simulink model "Impedance_with_fuzzy (1)"  (R2017b)
settings: Solver=ode45  StartTime=0.0  StopTime=20  RelTol=1e-3
libraries: cstblocks x1, fuzblock x1, simulink x1, commsrccod2 x1
settings Model: Creator=sansh  LastModifiedBy=pdesai24
settings CodeAppCC: StateflowObjectComments=on

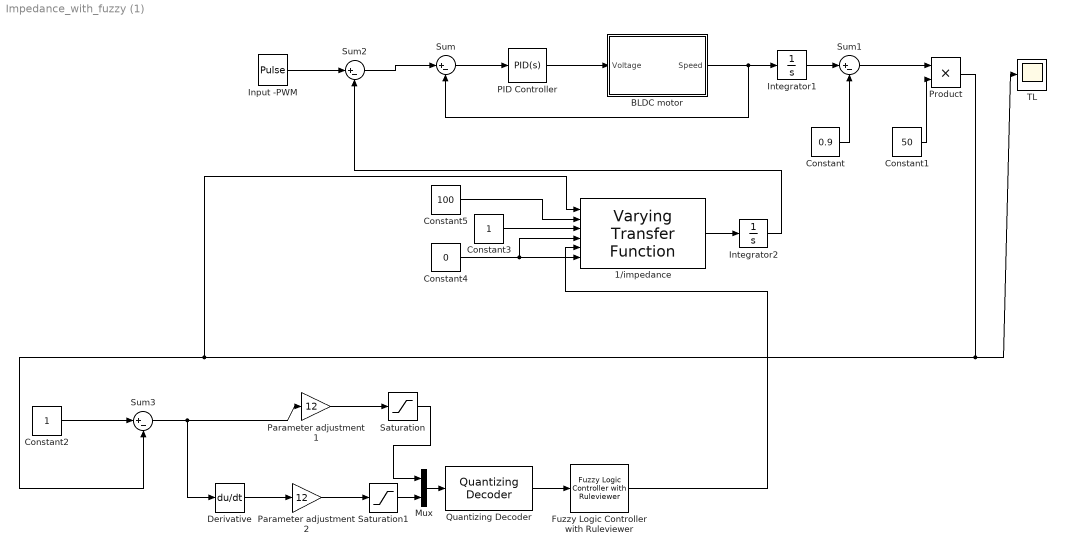
== system Impedance_with_fuzzy (1) ==
  1/impedance : cstblocks/Linear Parameter Varying/Varying Transfer Function  N=2
      settings: SourceProductName=Control System Toolbox
  BLDC motor : Subsystem
  Constant : Constant  Value=0.9
  Constant1 : Constant  Value=50
  Constant2 : Constant
  Constant3 : Constant
  Constant4 : Constant  Value=0
  Constant5 : Constant  Value=100
  Derivative : Derivative
  Fuzzy Logic Controller with Ruleviewer : fuzblock/Fuzzy Logic  Controller  with Ruleviewer  fismatrix=fuzzycntrl  Ts=2
  Input -PWM : DiscretePulseGenerator  PulseType=Time based  Amplitude=22  Period=10  PulseWidth=5  VectorParams1D=off
  Integrator1 : Integrator
  Integrator2 : Integrator
  Mux : Mux  Inputs=2
  PID Controller : simulink/Continuous/PID Controller  Controller=PID  TimeDomain=Continuous-time  SampleTime=-1  IntegratorMethod=Forward Euler  FilterMethod=Forward Euler  Form=Parallel  UseFilter=on  ControllerParametersSource=internal  P=5.19214898731134e-10  I=1.34591440829613e-14  D=4.45038743536682e-06  N=0.507796880153597  InitialConditionSource=internal  InitialConditionForIntegrator=0  InitialConditionForFilter=0  ExternalReset=none  LimitOutput=off  UpperSaturationLimit=inf  LowerSaturationLimit=-inf  LinearizeAsGain=on  AntiWindupMode=none  Kb=1  TrackingMode=off  Kt=1  PParamMin=[]  PParamMax=[]  IParamMin=[]  IParamMax=[]  DParamMin=[]  DParamMax=[]  NParamMin=[]  NParamMax=[]  KbParamMin=[]  KbParamMax=[]  KtParamMin=[]  KtParamMax=[]  POutMin=[]  POutMax=[]  IOutMin=[]  IOutMax=[]  DOutMin=[]  DOutMax=[]  NOutMin=[]  NOutMax=[]  KbOutMin=[]  KbOutMax=[]  KtOutMin=[]  KtOutMax=[]  IntegratorOutMin=[]  IntegratorOutMax=[]  FilterOutMin=[]  FilterOutMax=[]  SumOutMin=[]  SumOutMax=[]  SumI1OutMin=[]  SumI1OutMax=[]  SumI2OutMin=[]  SumI2OutMax=[]  SumI3OutMin=[]  SumI3OutMax=[]  SumDOutMin=[]  SumDOutMax=[]  SaturationOutMin=[]  SaturationOutMax=[]  IntegratorContinuousStateAttributes=''  IntegratorStateMustResolveToSignalObject=off  IntegratorRTWStateStorageClass=Auto  FilterContinuousStateAttributes=''  FilterStateMustResolveToSignalObject=off  FilterRTWStateStorageClass=Auto  DifferentiatorICPrevScaledInput=0  DifferentiatorOutMin=[]  DifferentiatorOutMax=[]  FilterDiffOutCoefMin=[]  FilterDiffOutCoefMax=[]  SumDenOutMin=[]  SumDenOutMax=[]  SumNumOutMin=[]  SumNumOutMax=[]  ReciprocalOutMin=[]  ReciprocalOutMax=[]  DivideOutMin=[]  DivideOutMax=[]  TunerSelectOption=Transfer Function Based (PID Tuner App)
  Parameter adjustment 1 : Gain  Gain=12
  Parameter adjustment 2 : Gain  Gain=12
  Product : Product
  Quantizing Decoder : commsrccod2/Quantizing Decoder  codebook=[-.825 -.5 0, .5 .825]  QuDType=double
      settings: SourceProductName=Communications Toolbox  SourceProductBaseCode=CM
  Saturation : Saturate
  Saturation1 : Saturate
  Sum{,1..3} (4 alike) : Sum  Inputs=|+-
  TL : Scope
  wires:
  Sum/1 -> PID Controller/1
  Integrator1/1 -> Sum1/1
  Constant/1 -> Sum1/2
  Constant1/1 -> Product/2
  Sum1/1 -> Product/1
  1/impedance/1 -> Integrator2/1
  Sum2/1 -> Sum/1
  Input -PWM/1 -> Sum2/1
  BLDC motor/1(Speed) -> Sum/2, Integrator1/1
  Mux/1 -> Quantizing Decoder/1
  Product/1 -> TL/1, 1/impedance/1, Sum3/2
  Integrator2/1 -> Sum2/2
  Parameter adjustment 1/1 -> Saturation/1
  Saturation/1 -> Mux/1
  Parameter adjustment 2/1 -> Saturation1/1
  Saturation1/1 -> Mux/2
  Derivative/1 -> Parameter adjustment 2/1
  Sum3/1 -> Derivative/1, Parameter adjustment 1/1
  Constant2/1 -> Sum3/1
  Quantizing Decoder/1 -> Fuzzy Logic Controller with Ruleviewer/1
  Fuzzy Logic Controller with Ruleviewer/1 -> 1/impedance/5
  Constant4/1 -> 1/impedance/6, 1/impedance/4
  Constant5/1 -> 1/impedance/2
  Constant3/1 -> 1/impedance/3
  PID Controller/1 -> BLDC motor/1(Voltage)

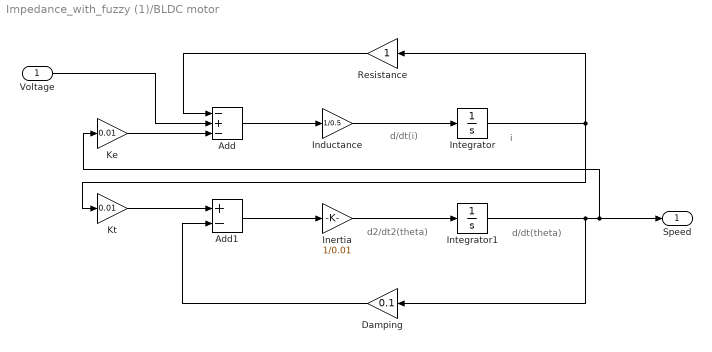
== system Impedance_with_fuzzy (1)/BLDC motor ==
  note: i
  note: d/dt(i)
  note: d/dt(theta)
  note: d2/dt2(theta)
  Voltage : Inport
  Add : Sum  Inputs=-+-
  Add1 : Sum  Inputs=+-
  Damping : Gain  Gain=0.1
  Inductance : Gain  Gain=1/0.5
  Inertia : Gain  Gain=1/0.01
  Integrator : Integrator
  Integrator1 : Integrator
  Ke : Gain  Gain=0.01
  Kt : Gain  Gain=0.01
  Resistance : Gain
  Speed : Outport
  wires:
  Inductance/1 -> Integrator/1
  Integrator1/1 -> Damping/1, Speed/1, Ke/1
  Inertia/1 -> Integrator1/1
  Integrator/1 -> Resistance/1, Kt/1
  Kt/1 -> Add1/1
  Voltage/1 -> Add/2
  Resistance/1 -> Add/1
  Damping/1 -> Add1/2
  Ke/1 -> Add/3
  Add/1 -> Inductance/1
  Add1/1 -> Inertia/1
